simulink model "sl_pursuit"  (R2015a)
settings: Solver=ode45  StartTime=0.0  StopTime=76  FixedStep=0.2  MaxStep=0.1  RelTol=1e-3
StartFcn:
  | % remove the red dashed line draw in StopFcn
  | h = findobj('Tag',  'SL_PURSUIT_PATH');
  | if ~isempty(h)
  |     delete(h)
  | end
StopFcn:
  | % get the waypoints from trajectory block
  | h = getSimulinkBlockHandle([gcs '/trajectory'])
  | path = str2num(get_param(h, 'path'));
  | 
  | % overlay it on the XY scope, tag it so it can be cleaned up in StartFcn
  | set(0, 'ShowHiddenHandles', 'on')
  | hold on
  | plot(path(:,1), path(:,2), 'Color',  'red', 'LineStyle', '--', 'LineWidth', 2, 'Tag', 'SL_PURSUIT_PATH')
  | hold off
  | set(0, 'ShowHiddenHandles', 'on')
libraries: roblocks x2, simulink x1, simulink_need_slupdate x1
settings Model: Creator=pic  LastModifiedBy=corkep
settings DataIOCC: LimitDataPoints=off  SignalLoggingSaveFormat=ModelDataLogs  ReturnWorkspaceOutputs=on  TimeSaveName=t  OutputSaveName=y
settings OptimizationCC: ExpressionDepthLimit=2147483647
settings DebuggingCC: UnderspecifiedInitializationDetection=Classic  MergeDetectMultiDrivingBlocksExec=none  SolverPrmCheckMsg=warning  FcnCallInpInsideContextMsg=EnableAllAsWarning  StateNameClashWarn=warning
settings GRTTargetCC: CombineOutputUpdateFcns=off  GRTInterface=on

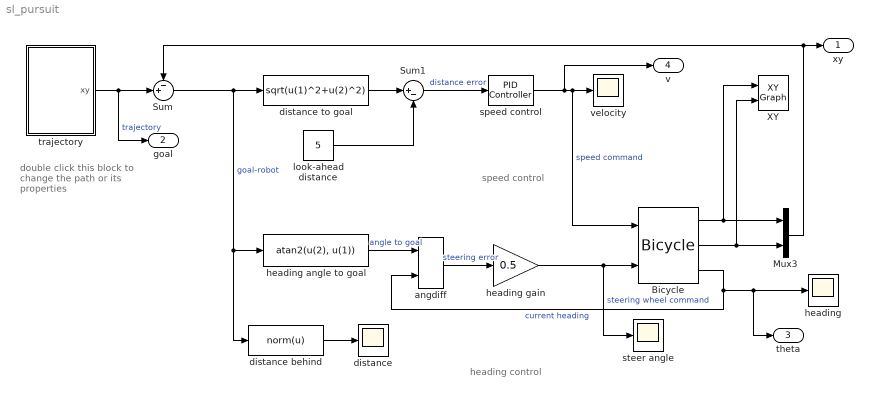
== system sl_pursuit ==
  note: speed control
  note: heading control
  note: double click this block to
      | change the path or its
      | properties
  Bicycle : roblocks/Vehicles/Bicycle  vlim=5  accel=1  alim=0.5  steer_rate=Inf  L=1  x0=[0, 0, 0]
  Mux3 : Mux  Inputs=2
  Sum : Sum  Inputs=-+|
  Sum1 : Sum  Inputs=|+-
  XY : simulink/Sinks/XY Graph  xmin=0  xmax=100  ymin=0  ymax=100  st=-1
  angdiff : roblocks/Toolbox/angdiff
  distance : Scope
      settings: TimeRange=auto  LimitDataPoints=on  MaxDataPoints=5000  SaveToWorkspace=off  SaveName=ScopeData3  YMin=0.79549  YMax=15.82273  SampleTime=-1
  distance behind : MATLABFcn  MATLABFcn=norm(u)
  distance to goal : Fcn  Expr=sqrt(u(1)^2+u(2)^2)
  "heading " : Scope
      settings: TimeRange=auto  LimitDataPoints=on  MaxDataPoints=5000  SaveToWorkspace=off  SaveName=ScopeData  YMin=-2.55814  YMax=2.03228  SampleTime=-1
  heading angle to goal : Fcn  Expr=atan2(u(2), u(1))
  heading gain : Gain  Gain=0.5
  look-ahead distance : Constant  Value=5
  speed control : simulink_need_slupdate/PID Controller  P=1  I=0.1  D=0
  steer angle : Scope
      settings: TimeRange=auto  LimitDataPoints=on  MaxDataPoints=5000  SaveToWorkspace=off  SaveName=ScopeData2  YMin=-0.67679  YMax=0.51839  SampleTime=-1
  trajectory : Subsystem  mask(Trajectory generator){path=|, vaxis=[2.5 2.5], tseg=[], dt=0.1, tacc=0, setsimtime=on}
      mask path=|
      | [  10 10;
      |   10 60;
      |   80 80;
      |   50 10 ]
      mask prompts: vaxis "Axis velocities"; tseg "Segment times"; dt "Sample interval"; tacc "Acceleration time"; setsimtime "Set Simulink simulation time"
      mask help: Generate an n-dimensional trajectory using the Toolbox function mstraj.
      mask init:
      | robot_traj = mstraj(path(2:end,:), vaxis, tseg, path(1,:), dt, tacc);
      | total_time = size(robot_traj,1)*dt;
      | if setsimtime
      |     set_param(gcs, 'StopTime', num2str(total_time));
      | end
      mask Help:
      | The trajectory requires a number of parameters
      | 
      | Path: an MxN matrix that defines a path with M points (start, intermediate, goal) and each point is defined by an N-dimensional vector.
      | 
      | Axis velocities: a 1xM vector that specifies the maximum speed of each motion for each dimension.
      | 
      | Segment times: a 1x(N-1) vector of times to execute each motion segment.
      | 
      | Sample time: a scalar sampling time, the trajectory is computed at discrete times with this separation.
      | 
      | Acceleration time: a scalar giving the period of acceleration at each waypoint, as the motion accelerates from one segment to the next.  Can be zero.
      | 
      | This block sets the Simulink simulation time to the length of the trajectory.
      mask Display: plot(path(:,1), path(:,2))
  velocity : Scope
      settings: TimeRange=auto  LimitDataPoints=on  MaxDataPoints=5000  SaveToWorkspace=off  YMin=-1.51264  YMax=10.52363  SampleTime=-1
  xy : Outport
  goal : Outport  Port=2
  theta : Outport  Port=3
  v : Outport  Port=4
  wires:
  Bicycle/1 -> Mux3/1, XY/1
  Bicycle/2 -> XY/2, Mux3/2
  Mux3/1 -> Sum/1, xy/1
  Sum/1 -> distance behind/1, heading angle to goal/1, distance to goal/1  "goal-robot"
  heading angle to goal/1 -> angdiff/1  "angle to goal"
  Bicycle/3 -> "heading "/1, theta/1, angdiff/2  "current heading"
  angdiff/1 -> heading gain/1  "steering error"
  heading gain/1 -> steer angle/1, Bicycle/2  "steering wheel command"
  speed control/1 -> Bicycle/1, velocity/1, v/1  "speed command"
  distance behind/1 -> distance/1
  trajectory/1(xy) -> goal/1, Sum/2  "trajectory"
  Sum1/1 -> speed control/1  "distance error"
  look-ahead distance/1 -> Sum1/2
  distance to goal/1 -> Sum1/1

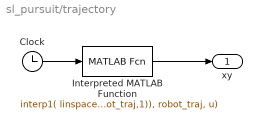
== system sl_pursuit/trajectory ==
  Clock : Clock
  Interpreted MATLAB Function : MATLABFcn  MATLABFcn=interp1( linspace(0, total_time, size(robot_traj,1)), robot_traj, u)
  xy : Outport
  wires:
  Clock/1 -> Interpreted MATLAB Function/1
  Interpreted MATLAB Function/1 -> xy/1
